simulink model "lab3_step_DM"  (R2019a)
settings: Solver=FixedStepAuto  StartTime=0.0  StopTime=10.0  RelTol=1e-3  EnableMultiTasking=on
undefined symbols (not defined in the file or in its folder): DiscIntNeverNeededParam
libraries: arduinolib x4
settings Model: ExtModeTrigDuration=2  Creator=MSI  LastModifiedBy=MSI
settings DataIOCC: ReturnWorkspaceOutputs=off
settings OptimizationCC: EnhancedBackFolding=on  PassReuseOutputArgsAs=Individual arguments  ZeroExternalMemoryAtStartup=off  ZeroInternalMemoryAtStartup=off  MaxStackSize=64  OptimizeBlockOrder=speed  DifferentSizesBufferReuse=on  OptimizationCustomize=off
settings DebuggingCC: ParameterTunabilityLossMsg=error  ArithmeticOperatorsInVariantConditions=warning
settings HardwareCC: ProdBitPerInt=16  ProdBitPerPointer=16  ProdBitPerSizeT=16  ProdBitPerPtrDiffT=16  ProdLargestAtomicFloat=None  ProdWordSize=8  ProdHWDeviceType=Atmel->AVR
settings SFSimCC: MATLABDynamicMemAlloc=off
settings RTWCC: SystemTargetFile=ert.tlc  HardwareBoard=Arduino Uno  TLCOptions=-aInlineSetEventsForThisBaseRateFcn=TLC_FALSE -aSuppressMultiTaskScheduler=TLC_FALSE -aRateBasedStepFcn=1  TemplateMakefile=ert_default_tmf  Toolchain=Arduino AVR  BuildConfiguration=Faster Runs
settings CodeAppCC: ForceParamTrailComments=on  IgnoreCustomStorageClasses=off  OperatorAnnotations=on  SimulinkDataObjDesc=on  SFDataObjDesc=on  InsertBlockDesc=on
settings ERTTargetCC: SupportContinuousTime=on  SupportVariableSizeSignals=on  ExtModeTransport=3  ExtModeStaticAlloc=on  ExtModeStaticAllocSize=250  ExtModeMexFile=ext_xcp  ExtModeIntrfLevel=Level2 - Open

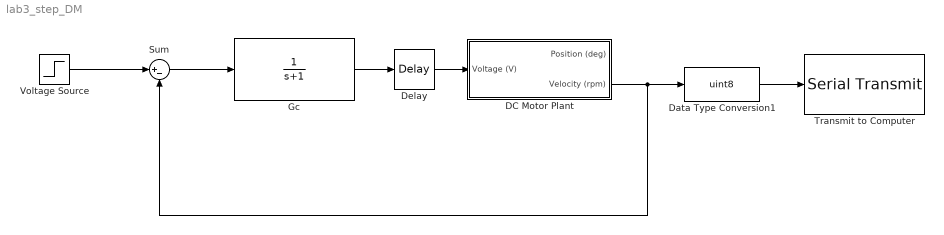
== system lab3_step_DM ==
  DC Motor Plant : Subsystem
  Data Type Conversion1 : DataTypeConversion  OutDataTypeStr=uint8  RndMeth=Round
  Delay : TransportDelay  DelayTime=0.01  BufferSize=128  FixedBuffer=on
  Gc : TransferFcn  Denominator=[1 1]
  Sum : Sum  Inputs=|+-
  Transmit to Computer : arduinolib/Serial Transmit  portNumber=0  sendmode=write  sendformat=Decimal  floatprecision=2  blockPlatform=arduino
  Voltage Source : Step  Time=0  After=40  SampleTime=0
  wires:
  Sum/1 -> Gc/1
  Voltage Source/1 -> Sum/1
  Data Type Conversion1/1 -> Transmit to Computer/1
  DC Motor Plant/2(Velocity (rpm)) -> Data Type Conversion1/1, Sum/2
  Gc/1 -> Delay/1
  Delay/1 -> DC Motor Plant/1(Voltage (V))

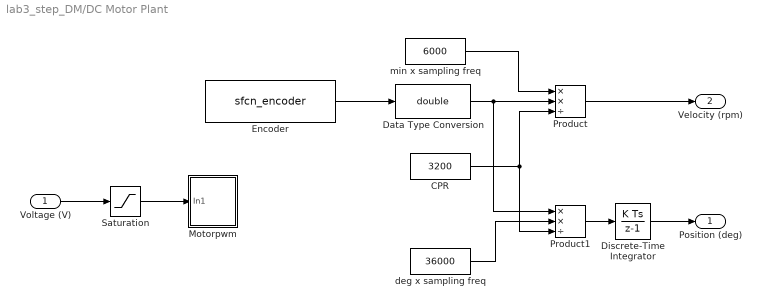
== system lab3_step_DM/DC Motor Plant ==
  Voltage (V) : Inport
  CPR : Constant  Value=3200
  Data Type Conversion : DataTypeConversion  OutDataTypeStr=double  RndMeth=Round
  Discrete-Time Integrator : DiscreteIntegrator  SampleTime=-1  ICPrevOutput=DiscIntNeverNeededParam  ICPrevScaledInput=DiscIntNeverNeededParam
  Encoder : S-Function  InitFcn=try, set_param(gcb,'FunctionName','sfcn_encoder'), end  FunctionName=sfcn_encoder  Parameters=uint8(0),uint8(2),uint8(3)  SFunctionModules=sfcn_encoder_wrapper  SFunctionDeploymentMode=off  EnableBusSupport=off  mask(S-Function Builder){}
      mask init:
      | val = [[.9  0.75 0.75 1 1 .9 .9 1]',[1 1 0.75 0.75 .9 .9 1 .9]'];try , sys = get_param(gcb,'SfunBuilderFcnName');if isempty(sys), sys = get_param(gcb,'FunctionName'); end,catch, sys = get_param(gcb,'FunctionName'); end
      settings: CopyFcn=set_param(gcbh,'LinkStatus','none')  PreSaveFcn=try, set_param(gcb,'FunctionName','sfcn_encoder'), end  OpenFcn=sfunctionwizard(gcbh)
      mask Display:
      | plot(val(:,1),val(:,2))
      | disp(sys)
      | port_label('output',1,'pos')
  Motorpwm : Subsystem
  Product : Product  Inputs=**/
  Product1 : Product  Inputs=**/
  Saturation : Saturate  UpperLimit=12  LowerLimit=-12
  deg x sampling freq : Constant  Value=36000
  min x sampling freq : Constant  Value=6000
  Position (deg) : Outport  VectorParamsAs1DForOutWhenUnconnected=off
  Velocity (rpm) : Outport  Port=2  VectorParamsAs1DForOutWhenUnconnected=off
  wires:
  CPR/1 -> Product1/3, Product/3
  Product/1 -> Velocity (rpm)/1
  Product1/1 -> Discrete-Time Integrator/1
  Encoder/1 -> Data Type Conversion/1
  Data Type Conversion/1 -> Product1/1, Product/2
  deg x sampling freq/1 -> Product1/2
  Voltage (V)/1 -> Saturation/1
  min x sampling freq/1 -> Product/1
  Saturation/1 -> Motorpwm/1(In1)
  Discrete-Time Integrator/1 -> Position (deg)/1

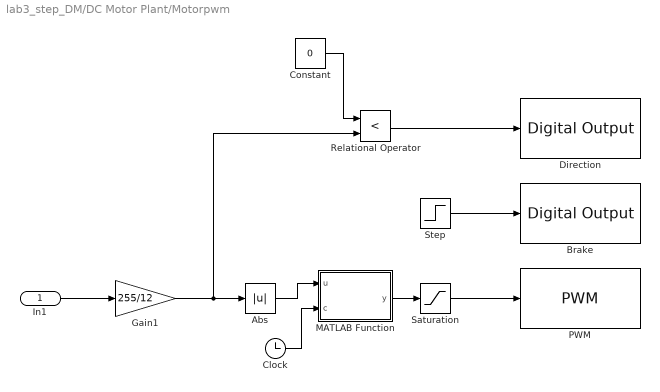
== system lab3_step_DM/DC Motor Plant/Motorpwm ==
  In1 : Inport
  Abs : Abs
  Brake : arduinolib/Digital Output  pinNumber=8  Direction=output  blockPlatform=arduino
  Clock : Clock
  Constant : Constant  Value=0
  "Direction " : arduinolib/Digital Output  pinNumber=13  Direction=output  blockPlatform=arduino
  Gain1 : Gain  Gain=255/12
  MATLAB Function : MATLAB Function  TreatAsAtomicUnit=on
  PWM : arduinolib/PWM  pinNumber=11  frequencyType=Default  desiredFrequency=490.2  achievableFrequency=490.2
  Relational Operator : RelationalOperator  Operator=<  OutDataTypeStr=boolean  RndMeth=Simplest
  Saturation : Saturate  UpperLimit=255  LowerLimit=0
  Step : Step  Time=0  After=0  SampleTime=0
  wires:
  Relational Operator/1 -> "Direction "/1
  Step/1 -> Brake/1
  Saturation/1 -> PWM/1
  In1/1 -> Gain1/1
  MATLAB Function/1(y) -> Saturation/1
  Abs/1 -> MATLAB Function/1(u)
  Clock/1 -> MATLAB Function/2(c)
  Gain1/1 -> Relational Operator/2, Abs/1
  Constant/1 -> Relational Operator/1

== matlab function lab3_step_DM/DC Motor Plant/Motorpwm/MATLAB Function ==
  data: u input; y output; c input
function y = fcn(u,c)
%#codegen
if c<10
    y = u;
else
    y=0;
end
